simulink library "BIO_TYPEA_MASTER"  (Simulink 8.6)
settings: Solver=ode45  StartTime=0.0  StopTime=10.0  RelTol=1e-3
libraries: STATE_BIO_MASTER x18
settings Model: Creator=controls  LastModifiedBy=controls

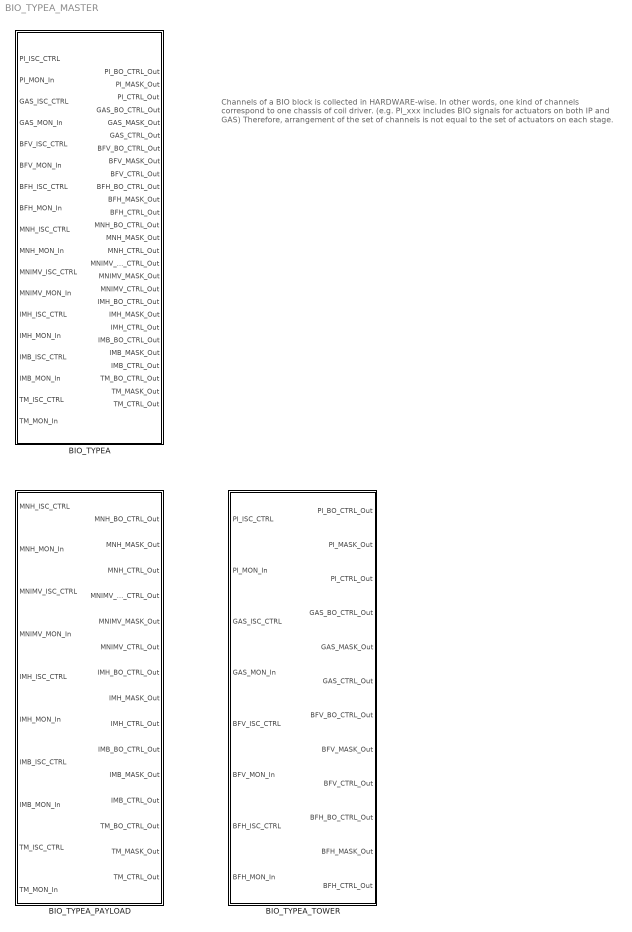
== system BIO_TYPEA_MASTER ==
  note: Channels of a BIO block is collected in HARDWARE-wise.
      | In other words, one kind of channels correspond to one chassis of coil driver.
      | (e.g. PI_xxx includes BIO signals for actuators on both IP and GAS)
      | Therefore, arrangement of the set of channels is not equal to the set of actuators on each stage.
  BIO_TYPEA : Subsystem
  BIO_TYPEA_PAYLOAD : Subsystem
  BIO_TYPEA_TOWER : Subsystem

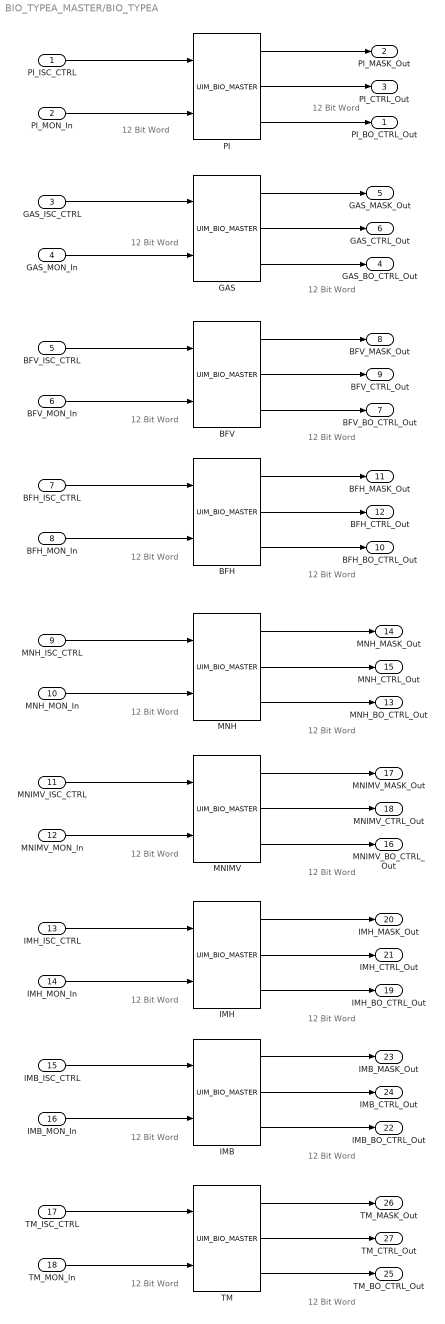
== system BIO_TYPEA_MASTER/BIO_TYPEA ==
  note: 12 Bit Word
  note: 12 Bit Word
  note: 12 Bit Word
  note: 12 Bit Word
  note: 12 Bit Word
  note: 12 Bit Word
  note: 12 Bit Word
  note: 12 Bit Word
  note: 12 Bit Word
  note: 12 Bit Word
  note: 12 Bit Word
  note: 12 Bit Word
  note: 12 Bit Word
  note: 12 Bit Word
  note: 12 Bit Word
  note: 12 Bit Word
  note: 12 Bit Word
  note: 12 Bit Word
  PI_ISC_CTRL : Inport
  PI_MON_In : Inport  Port=2
  GAS_ISC_CTRL : Inport  Port=3
  GAS_MON_In : Inport  Port=4
  BFV_ISC_CTRL : Inport  Port=5
  BFV_MON_In : Inport  Port=6
  BFH_ISC_CTRL : Inport  Port=7
  BFH_MON_In : Inport  Port=8
  MNH_ISC_CTRL : Inport  Port=9
  MNH_MON_In : Inport  Port=10
  MNIMV_ISC_CTRL : Inport  Port=11
  MNIMV_MON_In : Inport  Port=12
  IMH_ISC_CTRL : Inport  Port=13
  IMH_MON_In : Inport  Port=14
  IMB_ISC_CTRL : Inport  Port=15
  IMB_MON_In : Inport  Port=16
  TM_ISC_CTRL : Inport  Port=17
  TM_MON_In : Inport  Port=18
  BFH : STATE_BIO_MASTER/UIM_BIO_MASTER
  BFV : STATE_BIO_MASTER/UIM_BIO_MASTER
  GAS : STATE_BIO_MASTER/UIM_BIO_MASTER
  IMB : STATE_BIO_MASTER/UIM_BIO_MASTER
  IMH : STATE_BIO_MASTER/UIM_BIO_MASTER
  MNH : STATE_BIO_MASTER/UIM_BIO_MASTER
  MNIMV : STATE_BIO_MASTER/UIM_BIO_MASTER
  PI : STATE_BIO_MASTER/UIM_BIO_MASTER
  TM : STATE_BIO_MASTER/UIM_BIO_MASTER
  PI_BO_CTRL_Out : Outport
  PI_MASK_Out : Outport  Port=2
  PI_CTRL_Out : Outport  Port=3
  GAS_BO_CTRL_Out : Outport  Port=4
  GAS_MASK_Out : Outport  Port=5
  GAS_CTRL_Out : Outport  Port=6
  BFV_BO_CTRL_Out : Outport  Port=7
  BFV_MASK_Out : Outport  Port=8
  BFV_CTRL_Out : Outport  Port=9
  BFH_BO_CTRL_Out : Outport  Port=10
  BFH_MASK_Out : Outport  Port=11
  BFH_CTRL_Out : Outport  Port=12
  MNH_BO_CTRL_Out : Outport  Port=13
  MNH_MASK_Out : Outport  Port=14
  MNH_CTRL_Out : Outport  Port=15
  MNIMV_BO_CTRL_Out : Outport  Port=16
  MNIMV_MASK_Out : Outport  Port=17
  MNIMV_CTRL_Out : Outport  Port=18
  IMH_BO_CTRL_Out : Outport  Port=19
  IMH_MASK_Out : Outport  Port=20
  IMH_CTRL_Out : Outport  Port=21
  IMB_BO_CTRL_Out : Outport  Port=22
  IMB_MASK_Out : Outport  Port=23
  IMB_CTRL_Out : Outport  Port=24
  TM_BO_CTRL_Out : Outport  Port=25
  TM_MASK_Out : Outport  Port=26
  TM_CTRL_Out : Outport  Port=27
  wires:
  GAS_ISC_CTRL/1 -> GAS/1
  GAS_MON_In/1 -> GAS/2
  GAS/3 -> GAS_BO_CTRL_Out/1
  GAS/1 -> GAS_MASK_Out/1
  GAS/2 -> GAS_CTRL_Out/1
  PI_ISC_CTRL/1 -> PI/1
  PI_MON_In/1 -> PI/2
  PI/3 -> PI_BO_CTRL_Out/1
  PI/1 -> PI_MASK_Out/1
  PI/2 -> PI_CTRL_Out/1
  BFV_ISC_CTRL/1 -> BFV/1
  BFV_MON_In/1 -> BFV/2
  BFV/1 -> BFV_MASK_Out/1
  BFV/2 -> BFV_CTRL_Out/1
  BFV/3 -> BFV_BO_CTRL_Out/1
  MNH_ISC_CTRL/1 -> MNH/1
  MNH_MON_In/1 -> MNH/2
  MNH/1 -> MNH_MASK_Out/1
  MNH/2 -> MNH_CTRL_Out/1
  MNH/3 -> MNH_BO_CTRL_Out/1
  IMH_ISC_CTRL/1 -> IMH/1
  IMH_MON_In/1 -> IMH/2
  IMH/1 -> IMH_MASK_Out/1
  IMH/2 -> IMH_CTRL_Out/1
  IMH/3 -> IMH_BO_CTRL_Out/1
  TM_ISC_CTRL/1 -> TM/1
  TM_MON_In/1 -> TM/2
  TM/1 -> TM_MASK_Out/1
  TM/2 -> TM_CTRL_Out/1
  TM/3 -> TM_BO_CTRL_Out/1
  BFH_ISC_CTRL/1 -> BFH/1
  BFH_MON_In/1 -> BFH/2
  BFH/1 -> BFH_MASK_Out/1
  BFH/2 -> BFH_CTRL_Out/1
  BFH/3 -> BFH_BO_CTRL_Out/1
  MNIMV_ISC_CTRL/1 -> MNIMV/1
  MNIMV_MON_In/1 -> MNIMV/2
  MNIMV/1 -> MNIMV_MASK_Out/1
  MNIMV/2 -> MNIMV_CTRL_Out/1
  MNIMV/3 -> MNIMV_BO_CTRL_Out/1
  IMB_ISC_CTRL/1 -> IMB/1
  IMB_MON_In/1 -> IMB/2
  IMB/1 -> IMB_MASK_Out/1
  IMB/2 -> IMB_CTRL_Out/1
  IMB/3 -> IMB_BO_CTRL_Out/1

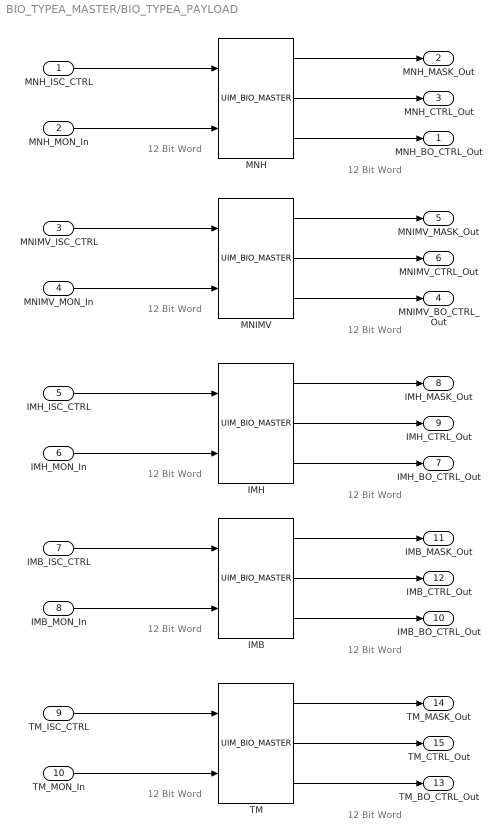
== system BIO_TYPEA_MASTER/BIO_TYPEA_PAYLOAD ==
  note: 12 Bit Word
  note: 12 Bit Word
  note: 12 Bit Word
  note: 12 Bit Word
  note: 12 Bit Word
  note: 12 Bit Word
  note: 12 Bit Word
  note: 12 Bit Word
  note: 12 Bit Word
  note: 12 Bit Word
  MNH_ISC_CTRL : Inport
  MNH_MON_In : Inport  Port=2
  MNIMV_ISC_CTRL : Inport  Port=3
  MNIMV_MON_In : Inport  Port=4
  IMH_ISC_CTRL : Inport  Port=5
  IMH_MON_In : Inport  Port=6
  IMB_ISC_CTRL : Inport  Port=7
  IMB_MON_In : Inport  Port=8
  TM_ISC_CTRL : Inport  Port=9
  TM_MON_In : Inport  Port=10
  IMB : STATE_BIO_MASTER/UIM_BIO_MASTER
  IMH : STATE_BIO_MASTER/UIM_BIO_MASTER
  MNH : STATE_BIO_MASTER/UIM_BIO_MASTER
  MNIMV : STATE_BIO_MASTER/UIM_BIO_MASTER
  TM : STATE_BIO_MASTER/UIM_BIO_MASTER
  MNH_BO_CTRL_Out : Outport
  MNH_MASK_Out : Outport  Port=2
  MNH_CTRL_Out : Outport  Port=3
  MNIMV_BO_CTRL_Out : Outport  Port=4
  MNIMV_MASK_Out : Outport  Port=5
  MNIMV_CTRL_Out : Outport  Port=6
  IMH_BO_CTRL_Out : Outport  Port=7
  IMH_MASK_Out : Outport  Port=8
  IMH_CTRL_Out : Outport  Port=9
  IMB_BO_CTRL_Out : Outport  Port=10
  IMB_MASK_Out : Outport  Port=11
  IMB_CTRL_Out : Outport  Port=12
  TM_BO_CTRL_Out : Outport  Port=13
  TM_MASK_Out : Outport  Port=14
  TM_CTRL_Out : Outport  Port=15
  wires:
  MNH_ISC_CTRL/1 -> MNH/1
  MNH_MON_In/1 -> MNH/2
  MNH/1 -> MNH_MASK_Out/1
  MNH/2 -> MNH_CTRL_Out/1
  MNH/3 -> MNH_BO_CTRL_Out/1
  IMH_ISC_CTRL/1 -> IMH/1
  IMH_MON_In/1 -> IMH/2
  IMH/1 -> IMH_MASK_Out/1
  IMH/2 -> IMH_CTRL_Out/1
  IMH/3 -> IMH_BO_CTRL_Out/1
  TM_ISC_CTRL/1 -> TM/1
  TM_MON_In/1 -> TM/2
  TM/1 -> TM_MASK_Out/1
  TM/2 -> TM_CTRL_Out/1
  TM/3 -> TM_BO_CTRL_Out/1
  MNIMV_ISC_CTRL/1 -> MNIMV/1
  MNIMV_MON_In/1 -> MNIMV/2
  MNIMV/1 -> MNIMV_MASK_Out/1
  MNIMV/2 -> MNIMV_CTRL_Out/1
  MNIMV/3 -> MNIMV_BO_CTRL_Out/1
  IMB_ISC_CTRL/1 -> IMB/1
  IMB_MON_In/1 -> IMB/2
  IMB/1 -> IMB_MASK_Out/1
  IMB/2 -> IMB_CTRL_Out/1
  IMB/3 -> IMB_BO_CTRL_Out/1

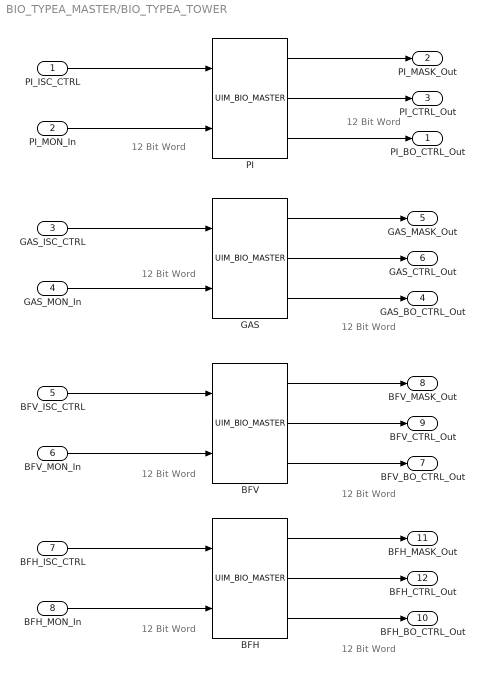
== system BIO_TYPEA_MASTER/BIO_TYPEA_TOWER ==
  note: 12 Bit Word
  note: 12 Bit Word
  note: 12 Bit Word
  note: 12 Bit Word
  note: 12 Bit Word
  note: 12 Bit Word
  note: 12 Bit Word
  note: 12 Bit Word
  PI_ISC_CTRL : Inport
  PI_MON_In : Inport  Port=2
  GAS_ISC_CTRL : Inport  Port=3
  GAS_MON_In : Inport  Port=4
  BFV_ISC_CTRL : Inport  Port=5
  BFV_MON_In : Inport  Port=6
  BFH_ISC_CTRL : Inport  Port=7
  BFH_MON_In : Inport  Port=8
  BFH : STATE_BIO_MASTER/UIM_BIO_MASTER
  BFV : STATE_BIO_MASTER/UIM_BIO_MASTER
  GAS : STATE_BIO_MASTER/UIM_BIO_MASTER
  PI : STATE_BIO_MASTER/UIM_BIO_MASTER
  PI_BO_CTRL_Out : Outport
  PI_MASK_Out : Outport  Port=2
  PI_CTRL_Out : Outport  Port=3
  GAS_BO_CTRL_Out : Outport  Port=4
  GAS_MASK_Out : Outport  Port=5
  GAS_CTRL_Out : Outport  Port=6
  BFV_BO_CTRL_Out : Outport  Port=7
  BFV_MASK_Out : Outport  Port=8
  BFV_CTRL_Out : Outport  Port=9
  BFH_BO_CTRL_Out : Outport  Port=10
  BFH_MASK_Out : Outport  Port=11
  BFH_CTRL_Out : Outport  Port=12
  wires:
  GAS_ISC_CTRL/1 -> GAS/1
  GAS_MON_In/1 -> GAS/2
  GAS/3 -> GAS_BO_CTRL_Out/1
  GAS/1 -> GAS_MASK_Out/1
  GAS/2 -> GAS_CTRL_Out/1
  PI_ISC_CTRL/1 -> PI/1
  PI_MON_In/1 -> PI/2
  PI/3 -> PI_BO_CTRL_Out/1
  PI/1 -> PI_MASK_Out/1
  PI/2 -> PI_CTRL_Out/1
  BFV_ISC_CTRL/1 -> BFV/1
  BFV_MON_In/1 -> BFV/2
  BFV/1 -> BFV_MASK_Out/1
  BFV/2 -> BFV_CTRL_Out/1
  BFV/3 -> BFV_BO_CTRL_Out/1
  BFH_ISC_CTRL/1 -> BFH/1
  BFH_MON_In/1 -> BFH/2
  BFH/1 -> BFH_MASK_Out/1
  BFH/2 -> BFH_CTRL_Out/1
  BFH/3 -> BFH_BO_CTRL_Out/1
